simulink model "LyFlow"  (R2018b)
settings: Solver=FixedStepDiscrete  StartTime=0.0  StopTime=10.0  FixedStep=0.01  RelTol=1e-3
settings Model: ModifiedHistory="2023.11.16  V2.3.0 Issue 566045 全躺，vip，腿托打开增加前后位置"  Creator=sn2xws  LastModifiedBy=sn2xws
settings DataIOCC: SaveFormat=StructureWithTime
settings OptimizationCC: DefaultParameterBehavior=Inlined  EnhancedBackFolding=on  PassReuseOutputArgsAs=Individual arguments  ZeroExternalMemoryAtStartup=off  ZeroInternalMemoryAtStartup=off  OptimizeBlockOrder=speed  DifferentSizesBufferReuse=on  OptimizationCustomize=off
settings DebuggingCC: ParameterTunabilityLossMsg=error
settings SFSimCC: MATLABDynamicMemAlloc=off
settings RTWCC: SystemTargetFile=autosar.tlc  GenCodeOnly=on  TemplateMakefile=ert_default_tmf  Description=AUTOSAR  GenerateReport=on  IncludeHyperlinkInReport=on  LaunchReport=on  GenerateTraceInfo=on  GenerateTraceReport=on  GenerateTraceReportSl=on  GenerateTraceReportSf=on  GenerateTraceReportEml=on  GenerateCodeMetricsReport=on
settings CodeAppCC: ForceParamTrailComments=on  IgnoreCustomStorageClasses=off  OperatorAnnotations=on  SimulinkDataObjDesc=on  SFDataObjDesc=on  InsertBlockDesc=on
settings STFCustomTargetCC: TargetLangStandard=C99 (ISO)  MultiwordLength=256  ParMdlRefBuildCompliant=on  CompOptLevelCompliant=on  IncludeMdlTerminateFcn=off  CombineOutputUpdateFcns=on  SuppressErrorStatus=on  ERTCustomFileBanners=on  SupportNonFinite=off  SupportComplex=off  SupportContinuousTime=off  SupportNonInlinedSFcns=off  RemoveResetFunc=on  MATLABClassNameForMDSCustomization=Simulink.SoftwareTarget.ERTCustomization  AutosarCompliant=on  UseToolchainInfoCompliant=on  LookupTableObjectStructAxisOrder=2,1,3,4,...  LUTObjectStructOrderEvenSpacing=Size,Table,Breakpoints  SystemTargetFile=autosar.tlc
settings ERTTargetCC: TargetLangStandard=C99 (ISO)  ConcurrentExecutionCompliant=off  IncludeMdlTerminateFcn=off  SuppressErrorStatus=on  SupportNonFinite=off  SupportComplex=off  ModelStepFunctionPrototypeControlCompliant=off  CPPClassGenCompliant=off  AutosarCompliant=on  LookupTableObjectStructAxisOrder=2,1,3,4,...  LUTObjectStructOrderEvenSpacing=Size,Table,Breakpoints  InlinedParameterPlacement=NonHierarchical  ERTCustomFileTemplate=example_file_process.tlc  ERTFilePackagingFormat=Compact

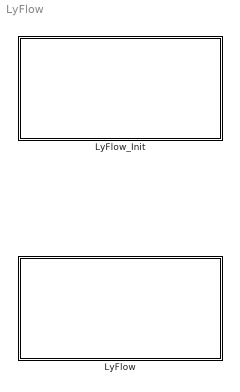
== system LyFlow ==
  LyFlow : Subsystem
  LyFlow_Init : Subsystem

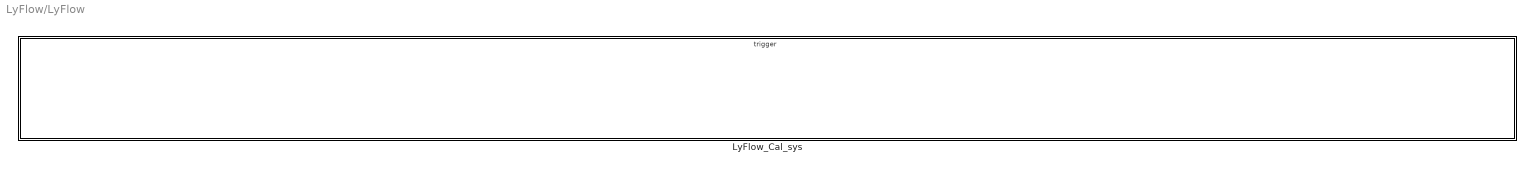
== system LyFlow/LyFlow ==
  LyFlow_Cal_sys : Subsystem

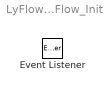
== system LyFlow/LyFlow_Init ==
  Event Listener : EventListener  EventName=reset

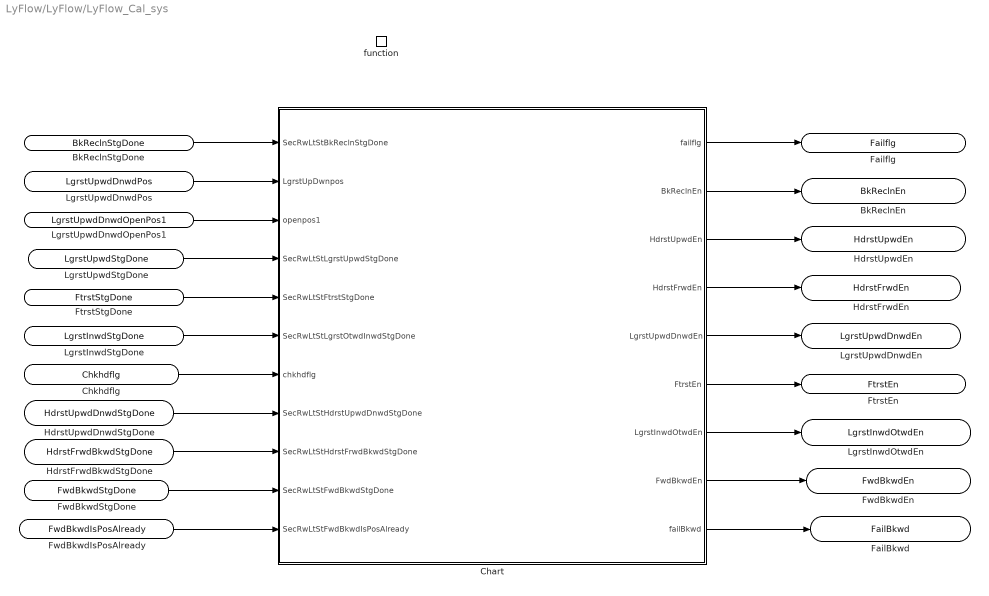
== system LyFlow/LyFlow/LyFlow_Cal_sys ==
  function : TriggerPort  TriggerType=function-call  IsSimulinkFunction=on  FunctionName=LyFlow_Cal  VariantControl=(inherit)
  Chart : Stateflow chart  TreatAsAtomicUnit=on
  BkReclnStgDone : ArgIn  OutDataTypeStr=boolean  ArgumentName=BkReclnStgDone
  LgrstUpwdDnwdPos : ArgIn  Port=2  OutDataTypeStr=uint16  ArgumentName=LgrstUpwdDnwdPos
  LgrstUpwdDnwdOpenPos1 : ArgIn  Port=3  OutDataTypeStr=uint16  ArgumentName=LgrstUpwdDnwdOpenPos1
  LgrstUpwdStgDone : ArgIn  Port=4  OutDataTypeStr=boolean  ArgumentName=LgrstUpwdStgDone
  FtrstStgDone : ArgIn  Port=5  OutDataTypeStr=boolean  ArgumentName=FtrstStgDone
  LgrstInwdStgDone : ArgIn  Port=6  OutDataTypeStr=boolean  ArgumentName=LgrstInwdStgDone
  Chkhdflg : ArgIn  Port=7  OutDataTypeStr=boolean  ArgumentName=Chkhdflg
  HdrstUpwdDnwdStgDone : ArgIn  Port=8  OutDataTypeStr=boolean  ArgumentName=HdrstUpwdDnwdStgDone
  HdrstFrwdBkwdStgDone : ArgIn  Port=9  OutDataTypeStr=boolean  ArgumentName=HdrstFrwdBkwdStgDone
  FwdBkwdStgDone : ArgIn  Port=10  OutDataTypeStr=boolean  ArgumentName=FwdBkwdStgDone
  FwdBkwdIsPosAlready : ArgIn  Port=11  OutDataTypeStr=boolean  ArgumentName=FwdBkwdIsPosAlready
  Failflg : ArgOut  OutDataTypeStr=boolean  ArgumentName=Failflg
  BkReclnEn : ArgOut  Port=2  OutDataTypeStr=boolean  ArgumentName=BkReclnEn
  HdrstUpwdEn : ArgOut  Port=3  OutDataTypeStr=boolean  ArgumentName=HdrstUpwdEn
  HdrstFrwdEn : ArgOut  Port=4  OutDataTypeStr=boolean  ArgumentName=HdrstFrwdEn
  LgrstUpwdDnwdEn : ArgOut  Port=5  OutDataTypeStr=boolean  ArgumentName=LgrstUpwdDnwdEn
  FtrstEn : ArgOut  Port=6  OutDataTypeStr=boolean  ArgumentName=FtrstEn
  LgrstInwdOtwdEn : ArgOut  Port=7  OutDataTypeStr=boolean  ArgumentName=LgrstInwdOtwdEn
  FwdBkwdEn : ArgOut  Port=8  OutDataTypeStr=boolean  ArgumentName=FwdBkwdEn
  FailBkwd : ArgOut  Port=9  OutDataTypeStr=boolean  ArgumentName=FailBkwd
  wires:
  BkReclnStgDone/1 -> Chart/1(SecRwLtStBkReclnStgDone)
  LgrstUpwdDnwdPos/1 -> Chart/2(LgrstUpDwnpos)
  LgrstUpwdDnwdOpenPos1/1 -> Chart/3(openpos1)
  LgrstUpwdStgDone/1 -> Chart/4(SecRwLtStLgrstUpwdStgDone)
  FtrstStgDone/1 -> Chart/5(SecRwLtStFtrstStgDone)
  LgrstInwdStgDone/1 -> Chart/6(SecRwLtStLgrstOtwdInwdStgDone)
  Chkhdflg/1 -> Chart/7(chkhdflg)
  HdrstUpwdDnwdStgDone/1 -> Chart/8(SecRwLtStHdrstUpwdDnwdStgDone)
  HdrstFrwdBkwdStgDone/1 -> Chart/9(SecRwLtStHdrstFrwdBkwdStgDone)
  Chart/1(failflg) -> Failflg/1
  Chart/2(BkReclnEn) -> BkReclnEn/1
  Chart/3(HdrstUpwdEn) -> HdrstUpwdEn/1
  Chart/4(HdrstFrwdEn) -> HdrstFrwdEn/1
  Chart/5(LgrstUpwdDnwdEn) -> LgrstUpwdDnwdEn/1
  Chart/6(FtrstEn) -> FtrstEn/1
  Chart/7(LgrstInwdOtwdEn) -> LgrstInwdOtwdEn/1
  Chart/8(FwdBkwdEn) -> FwdBkwdEn/1
  FwdBkwdStgDone/1 -> Chart/10(SecRwLtStFwdBkwdStgDone)
  FwdBkwdIsPosAlready/1 -> Chart/11(SecRwLtStFwdBkwdIsPosAlready)
  Chart/9(failBkwd) -> FailBkwd/1

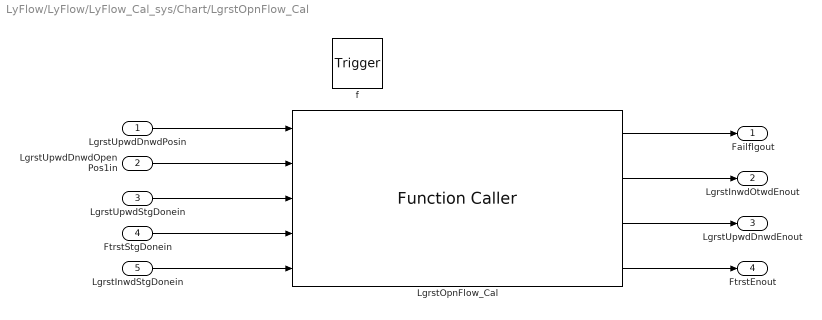
== system LyFlow/LyFlow/LyFlow_Cal_sys/Chart/LgrstOpnFlow_Cal ==
  LgrstUpwdDnwdPosin : Inport
  LgrstUpwdDnwdOpenPos1in : Inport  Port=2
  LgrstUpwdStgDonein : Inport  Port=3
  FtrstStgDonein : Inport  Port=4
  LgrstInwdStgDonein : Inport  Port=5
  f : TriggerPort  TriggerType=function-call  VariantControl=(inherit)
      settings: CopyFcn=Stateflow.SLINSF.SimulinkMan.removeBlockPreDeleteFcn  PreDeleteFcn=Stateflow.SLINSF.SimulinkMan.unsafePredeleteFcn
  LgrstOpnFlow_Cal : FunctionCaller  FunctionPrototype=[Failflg,LgrstInwdOtwdEn,LgrstUpwdDnwdEn,FtrstEn] = LgrstOpnFlow_Cal(LgrstUpwdDnwdPos,LgrstUpwdDnwdOpenPos1,LgrstUpwdStgDone,FtrstStgDone,LgrstInwdStgDone)  InputArgumentSpecifications=uint16(1), uint16(1), boolean(true), boolean(true), boolean(true)  OutputArgumentSpecifications=boolean(true), boolean(true), boolean(true), boolean(true)
  Failflgout : Outport
  LgrstInwdOtwdEnout : Outport  Port=2
  LgrstUpwdDnwdEnout : Outport  Port=3
  FtrstEnout : Outport  Port=4
  wires:
  LgrstOpnFlow_Cal/2 -> LgrstInwdOtwdEnout/1
  LgrstOpnFlow_Cal/1 -> Failflgout/1
  LgrstOpnFlow_Cal/3 -> LgrstUpwdDnwdEnout/1
  LgrstOpnFlow_Cal/4 -> FtrstEnout/1
  LgrstUpwdDnwdPosin/1 -> LgrstOpnFlow_Cal/1
  LgrstUpwdDnwdOpenPos1in/1 -> LgrstOpnFlow_Cal/2
  LgrstUpwdStgDonein/1 -> LgrstOpnFlow_Cal/3
  FtrstStgDonein/1 -> LgrstOpnFlow_Cal/4
  LgrstInwdStgDonein/1 -> LgrstOpnFlow_Cal/5

== stateflow chart LyFlow/LyFlow_Cal_sys/Chart ==
  state [Failflgout,LgrstInwdOtwdEnout,LgrstUpwdDnwdEnout,FtrstEnout] = LgrstOpnFlow_Cal(LgrstUpwdDnwdPosin,LgrstUpwdDnwdOpenPos1in,LgrstUpwdStgDonein,FtrstStgDonein,LgrstInwdStgDonein) [function]
  note: 2023.11.16 V2.3.0 Issue 566045 全躺，vip，腿托打开增加前后位置
  (default) -> (junction 224) : {
      | failflg =0;
      | BkReclnEn=0;
      | HdrstUpwdEn=0;
      | HdrstFrwdEn=0;
      | LgrstUpwdDnwdEn=0;
      | FtrstEn=0;
      | LgrstInwdOtwdEn=0;
      | FwdBkwdEn = 0;
      | failBkwd=0;
      | }
  (junction 224) -> (junction 231) [order 1] : [!SecRwLtStFwdBkwdStgDone]
  (junction 224) -> (junction 236) [order 2]
  (junction 231) -> (junction 241) : {FwdBkwdEn=1;}
  (junction 236) -> (junction 244) [order 1] : [!SecRwLtStFwdBkwdIsPosAlready]
  (junction 236) -> (junction 5) [order 2]
  (junction 244) -> (junction 245) : {failBkwd=1;}
  (junction 241) -> (junction 247)
  (junction 245) -> (junction 247)
  (junction 247) -> (junction 173)
  (junction 5) -> (junction 9) [order 1] : [SecRwLtStBkReclnStgDone]
  (junction 5) -> (junction 7) [order 2] : {
      | BkReclnEn=1;
      | }
  (junction 9) -> (junction 11)
  (junction 11) -> (junction 7)
  (junction 7) -> (junction 183) : {[failflg,LgrstInwdOtwdEn,LgrstUpwdDnwdEn,FtrstEn] = LgrstOpnFlow_Cal(LgrstUpDwnpos,openpos1,SecRwLtStLgrstUpwdStgDone,SecRwLtStFtrstStgDone,SecRwLtStLgrstOtwdInwdStgDone);}
  (junction 183) -> (junction 125)
  (junction 125) -> (junction 134) [order 1] : [(SecRwLtStLgrstUpwdStgDone&&SecRwLtStFtrstStgDone&&SecRwLtStLgrstOtwdInwdStgDone)||...
      | failflg]
  (junction 134) -> (junction 136) [order 1] : [chkhdflg]
  (junction 136) -> (junction 168) [order 1] : [SecRwLtStHdrstUpwdDnwdStgDone]
  (junction 168) -> (junction 173) [order 1] : [SecRwLtStHdrstFrwdBkwdStgDone]
  (junction 125) -> (junction 128) [order 2]
  (junction 134) -> (junction 140) [order 2]
  (junction 136) -> (junction 170) [order 2] : {
      | HdrstUpwdEn=1;
      | }
  (junction 168) -> (junction 178) [order 2] : {
      | HdrstFrwdEn=1;
      | }
  (junction 173) -> (junction 175)
  (junction 140) -> (junction 142) [order 1] : [SecRwLtStHdrstUpwdDnwdStgDone]
  (junction 140) -> (junction 151) [order 2] : {
      | HdrstUpwdEn=1;
      | }
  (junction 142) -> (junction 149)
  (junction 149) -> (junction 151)
  (junction 151) -> (junction 154)
  (junction 154) -> (junction 156) [order 1] : [SecRwLtStHdrstFrwdBkwdStgDone]
  (junction 154) -> (junction 160) [order 2] : {
      | HdrstFrwdEn=1;
      | }
  (junction 156) -> (junction 158)
  (junction 158) -> (junction 160)
  (junction 160) -> (junction 163)
  (junction 163) -> (junction 128)
  (junction 170) -> (junction 163)
  (junction 178) -> (junction 170)
  (junction 175) -> (junction 178)
  (junction 128) -> (junction 166)
  data: LgrstUpwdDnwdPosin function_input; LgrstUpwdDnwdOpenPos1in function_input; LgrstUpwdStgDonein function_input; FtrstStgDonein function_input; LgrstInwdStgDonein function_input; Failflgout function_output; LgrstInwdOtwdEnout function_output; LgrstUpwdDnwdEnout function_output; FtrstEnout function_output; SecRwLtStBkReclnStgDone input boolean; LgrstUpDwnpos input uint16; openpos1 input uint16; SecRwLtStLgrstUpwdStgDone input boolean; SecRwLtStFtrstStgDone input boolean; SecRwLtStLgrstOtwdInwdStgDone input boolean; chkhdflg input boolean; SecRwLtStHdrstUpwdDnwdStgDone input boolean; SecRwLtStHdrstFrwdBkwdStgDone input boolean; failflg output boolean; BkReclnEn output boolean; HdrstUpwdEn output boolean; HdrstFrwdEn output boolean; LgrstUpwdDnwdEn output boolean; FtrstEn output boolean; LgrstInwdOtwdEn output boolean; FwdBkwdEn output boolean; SecRwLtStFwdBkwdStgDone input boolean; SecRwLtStFwdBkwdIsPosAlready input boolean; failBkwd output boolean
